simulink library "MedusaDrHoligramEq"  (R2022b)
settings: Solver=VariableStepAuto  StartTime=0.0  StopTime=10.0  RelTol=1e-3
undefined symbols (not defined in the file or in its folder): Row
libraries: TuneVar x6, TOP x3, HandyTextFile x2, FeaturePath x1, FirGeneric x1, PoolIir x1
settings Model: Creator=ud1041536  LastModifiedBy=sc48041
settings SolverCC: AlgebraicLoopSolver=TrustRegion
settings DebuggingCC: UnconnectedInputMsg=warning  UnconnectedOutputMsg=warning  UnconnectedLineMsg=warning  SFMachineParentedDataDiag=warning  ArithmeticOperatorsInVariantConditions=warning
settings ModelReferenceCC: EnableRefExpFcnMdlSchedulingChecks=on
settings SFSimCC: CustomCodeUndefinedFunction=UseInterfaceOnly

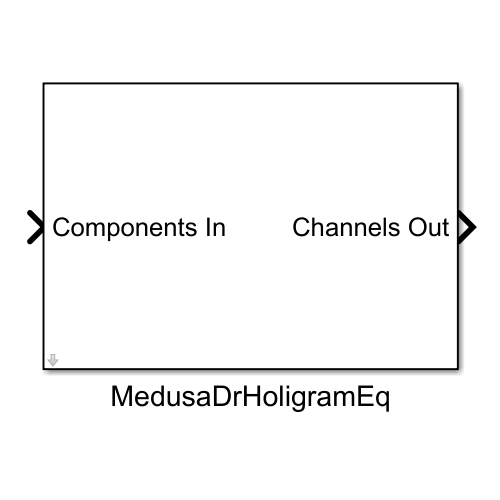
[thumbnail: Simulink's stored preview of the top-level diagram]
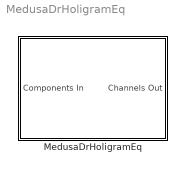
== system MedusaDrHoligramEq ==
  MedusaDrHoligramEq : Subsystem  mask{Config=[]}
      mask prompts: Config "MedusaDrHoligramEqConfig"
      mask init:
      | blkh=gcbh;
      | Config=BTConfig.Assert(blkh,Config);
      | 
      | Config.Validate();
      | Config.DoMaskInit(blkh);

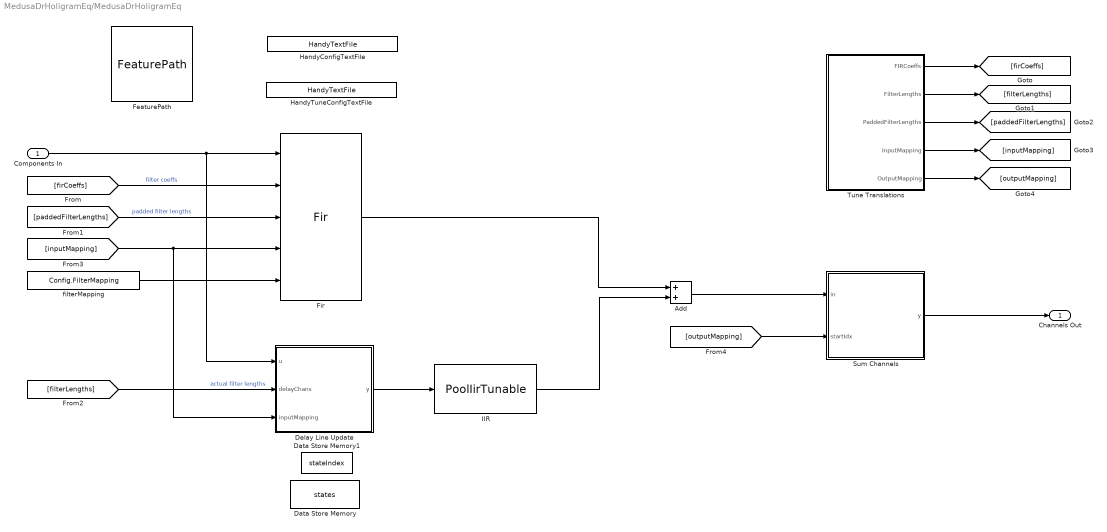
== system MedusaDrHoligramEq/MedusaDrHoligramEq ==
  Components In : Inport
  Add : Sum  Priority=2
  Data Store Memory : DataStoreMemory  DataStoreName=states  ReadBeforeWriteMsg=warning  WriteAfterWriteMsg=warning  WriteAfterReadMsg=warning  InitialValue=Config.DelayStateInitVal  ShowAdditionalParam=off  OutDataTypeStr=single
  Data Store Memory1 : DataStoreMemory  DataStoreName=stateIndex  ReadBeforeWriteMsg=warning  WriteAfterWriteMsg=warning  WriteAfterReadMsg=warning  ShowAdditionalParam=off  OutDataTypeStr=int32
  Delay Line Update : MATLAB Function  TreatAsAtomicUnit=on  mask{fixedDelayLength=Config.FixedDelayLength}
  FeaturePath : FeaturePath/FeaturePath  FeatureName=DRHoligram  IsGroup=off  GroupNumber=-1  IsModule=off  TriggerInit=[375 434 490 541]
      settings: SourceProductName=Bose Talaria
  Fir : FirGeneric/Fir  Config=Config.Fir
      settings: SourceProductName=Bose Blocklib
  HandyConfigTextFile : HandyTextFile/HandyTextFile  TemplateSource=Config  FileSuffix=File  OpenDialogOnLoad=off  UseThisBlockName=off  AddGrandParentNamePrefix=off  TheDefaultText=% $(FILENAME) $(PREFIX) $(SUFFIX)  ShowInLibBrowser=on
      settings: SourceProductName=Bose Talaria
  HandyTuneConfigTextFile : HandyTextFile/HandyTextFile  TemplateSource=TuneConfig  FileSuffix=File  OpenDialogOnLoad=off  UseThisBlockName=off  AddGrandParentNamePrefix=off  TheDefaultText=% $(FILENAME) $(PREFIX) $(SUFFIX)  ShowInLibBrowser=on
      settings: SourceProductName=Bose Talaria
  IIR : PoolIir/PoolIirTunable  FeatureName=PoolIirTunableConfig  Config=Config.Iir
  Sum Channels : MATLAB Function  Priority=3  TreatAsAtomicUnit=on
  Tune Translations : Subsystem
  filterMapping : Constant  Value=Config.FilterMapping  VectorParams1D=off  OutDataTypeStr=uint32
  Channels Out : Outport  VectorParamsAs1DForOutWhenUnconnected=off
  wires:
  Sum Channels/1(y) -> Channels Out/1
  IIR/1 -> Add/2
  filterMapping/1 -> Fir/5
  Delay Line Update/1(y) -> IIR/1
  Add/1 -> Sum Channels/1(in)
  [outputMapping] -> Sum Channels/2(startIdx)
  [inputMapping] -> Fir/4, Delay Line Update/3(inputMapping)
  Components In/1 -> Delay Line Update/1(u), Fir/1
  [filterLengths] -> Delay Line Update/2(delayChans)  "actual filter lengths"
  Tune Translations/1(FIRCoeffs) -> [firCoeffs]
  Tune Translations/2(FilterLengths) -> [filterLengths]
  Tune Translations/3(PaddedFilterLengths) -> [paddedFilterLengths]
  Tune Translations/4(InputMapping) -> [inputMapping]
  Tune Translations/5(OutputMapping) -> [outputMapping]
  Fir/1 -> Add/1
  [firCoeffs] -> Fir/2  "filter coeffs"
  [paddedFilterLengths] -> Fir/3  "padded filter lengths"

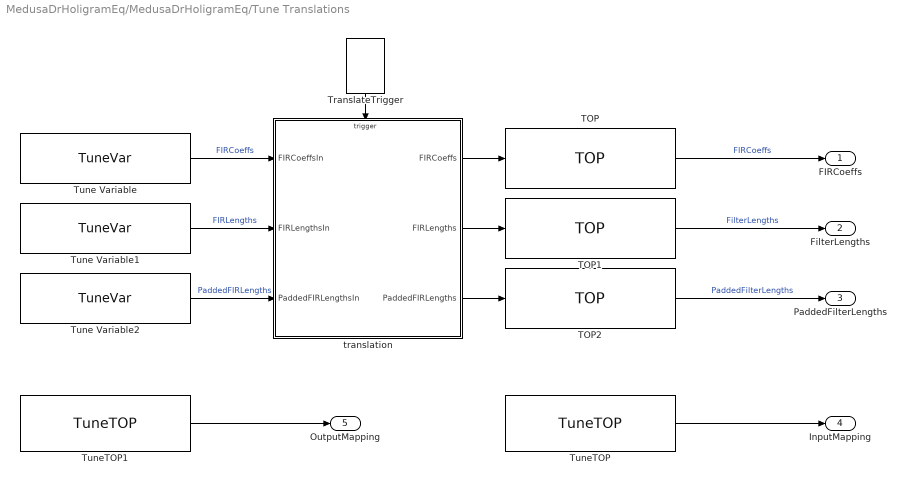
== system MedusaDrHoligramEq/MedusaDrHoligramEq/Tune Translations ==
  TOP : TOP/TOP  TriggerInit=[815 200 985 260]  TopName=FIRCoeffs  DataTypeOut=single  BankNumber=1  PreOverlay=false  PostOverlay=false  Role=Automatic
      settings: SourceProductName=Bose Talaria
  TOP1 : TOP/TOP  TriggerInit=[815 270 985 330]  TopName=FilterLengths  DataTypeOut=uint32  BankNumber=0  PreOverlay=false  PostOverlay=false  Role=Automatic
      settings: SourceProductName=Bose Talaria
  TOP2 : TOP/TOP  TriggerInit=[815 340 985 400]  TopName=PaddedFilterLengths  DataTypeOut=uint32  BankNumber=0  PreOverlay=false  PostOverlay=false  Role=Automatic
      settings: SourceProductName=Bose Talaria
  TranslateTrigger : TuneVar/TranslateTrigger  TriggerInit=[656 110 694 165]
      settings: SourceProductName=Bose Talaria
  Tune Variable : TuneVar/TuneVar  TuneName=FIRCoeffs  SpecifyMaxSize=off  VariableDim=1 (Row)  MaxSize=[Config.AvgFirLength*Config.TotalNumEqLinks 1]  TunabilityNumber=1  MinValue=[]  MaxValue=[]  TriggerInit=[20 115 190 165]  MaskValue=Config.TuneDefaults.FirCoeffs
      settings: SourceProductName=Bose Talaria
  Tune Variable1 : TuneVar/TuneVar  TuneName=FIRLengths  SpecifyMaxSize=off  VariableDim=1 (Row)  MaxSize=[1 1]  TunabilityNumber=1  MinValue=[]  MaxValue=[]  TriggerInit=[20 185 190 235]  MaskValue=Config.TuneDefaults.FirLengths
      settings: SourceProductName=Bose Talaria
  Tune Variable2 : TuneVar/TuneVar  TuneName=PaddedFIRLengths  SpecifyMaxSize=off  VariableDim=1 (Row)  MaxSize=[1 1]  TunabilityNumber=1  MinValue=[]  MaxValue=[]  TriggerInit=[20 255 190 305]  MaskValue=Config.TuneDefaults.PaddedFirLengths
      settings: SourceProductName=Bose Talaria
  TuneTOP : TuneVar/TuneTOP  TriggerInit=[505 377 675 433]  TopName=InputMapping  TuneName=InputMapping  DataTypeOut=uint32  TunabilityNumber=1  MinValue=[]  MaxValue=[]  BankNumber=0  PreOverlay=false  PostOverlay=false  UseSameName=on  MaskValue=Config.TuneDefaults.InputMapping
      settings: SourceProductName=Bose Talaria
  TuneTOP1 : TuneVar/TuneTOP  TriggerInit=[20 377 190 433]  TopName=OutputMapping  TuneName=OutputMapping  DataTypeOut=single  TunabilityNumber=1  MinValue=[]  MaxValue=[]  BankNumber=0  PreOverlay=false  PostOverlay=false  UseSameName=on  MaskValue=Config.TuneDefaults.OutputMapping
      settings: SourceProductName=Bose Talaria
  translation : MATLAB Function  TreatAsAtomicUnit=on
  FIRCoeffs : Outport
  FilterLengths : Outport  Port=2
  PaddedFilterLengths : Outport  Port=3
  InputMapping : Outport  Port=4
  OutputMapping : Outport  Port=5
  wires:
  Tune Variable2/1 -> translation/3(PaddedFIRLengthsIn)  "PaddedFIRLengths"
  translation/2(FIRLengths) -> TOP1/1
  TuneTOP1/1 -> OutputMapping/1
  Tune Variable/1 -> translation/1(FIRCoeffsIn)  "FIRCoeffs"
  Tune Variable1/1 -> translation/2(FIRLengthsIn)  "FIRLengths"
  translation/3(PaddedFIRLengths) -> TOP2/1
  TuneTOP/1 -> InputMapping/1
  translation/1(FIRCoeffs) -> TOP/1
  TranslateTrigger/1 -> translation/Trigger
  TOP1/1 -> FilterLengths/1  "FilterLengths"
  TOP/1 -> FIRCoeffs/1  "FIRCoeffs"
  TOP2/1 -> PaddedFilterLengths/1  "PaddedFilterLengths"

== matlab function MedusaDrHoligramEq/Delay Line Update ==
  data: u input; y output; delayChans input; inputMapping input; states data_store_memory; stateIndex data_store_memory; fixedDelayLength parameter
function y = delayLineUpdate(u, delayChans, inputMapping, fixedDelayLength)

% Note: This block only reads 'states' to get the delayed samples. A
% separate function is responsible for writing to 'states' to update the 
% delay line Data Store Memory. Thus it is important to ensure all DSM  
% write happens before DSM read.
%
% This is different from pooldelay, as the delay for ALL channel is
% intentionally set to be the max amount to allow for 'double' sharing
% between FIR filter and delay buffer.

global states;
global stateIndex; 

numOutput = numel(delayChans);
[frameSize, numChannelIn] = size(u);
y = single(zeros(frameSize, numOutput));
delayChans = int32(delayChans);

% Write incoming input to delay line
writeIdx = stateIndex;
for sample = 1:frameSize
    for i = 1:numChannelIn
        states(writeIdx+1,i) = u(sample, i); % add 1 for Matlab indexing
    end
    writeIdx = circindex(writeIdx, int32(1), fixedDelayLength);
end
stateIndex = writeIdx;

% Read out values from delay line
for i = 1:numOutput
    inputIdx = inputMapping(i);  % which input to delay
    delay = delayChans(i);       % delay amount
    offset = - (delay + frameSize); % offset from start index
    readIdx = circindex(stateIndex, offset, fixedDelayLength);
    
    for sample = 1:frameSize
        y(sample, i) = states(readIdx+1, inputIdx+1); % add 1 for Matlab indexing
        readIdx = circindex(readIdx, int32(1), fixedDelayLength);
    end
end

== matlab function MedusaDrHoligramEq/Sum Channels ==
  data: in input; y output; startIdx input
function y = sum_channels(in, startIdx)
[frame_size, ~] = size(in);
[num_output, ~] = size(startIdx);

y = coder.nullcopy(single(zeros(frame_size, num_output)));
for iter = 1:num_output-1
    start_idx = startIdx(iter);
    end_idx = startIdx(iter+1)-1;
    y(:,iter) = sum(in(:,start_idx+1:end_idx+1),2);
end
start_idx = startIdx(end);
y(:,end) = sum(in(:,start_idx+1:end),2);

== matlab function MedusaDrHoligramEq/Tune Translations/translation ==
  data: FIRCoeffs output; FIRCoeffsIn input; FIRLengths output; FIRLengthsIn input; PaddedFIRLengthsIn input; PaddedFIRLengths output
  events: trigger input FUNCTION_CALL_EVENT
function [FIRCoeffs, FIRLengths, PaddedFIRLengths] = fcn(FIRCoeffsIn, FIRLengthsIn, PaddedFIRLengthsIn)

FIRCoeffs = FIRCoeffsIn.Value;
FIRLengths = FIRLengthsIn.Value;
PaddedFIRLengths = PaddedFIRLengthsIn.Value;
